simulink model "hexGroundContact"  (R2024a)
settings: configuration reference "standardSILConfiguraitonParams" (kept outside this file)
libraries: matrix_library x3, simulink x1
settings Model: Creator=jerem  LastModifiedBy=jerem
settings ConfigSetRef: SourceName=standardSILConfiguraitonParams  SourceLocation=Base Workspace

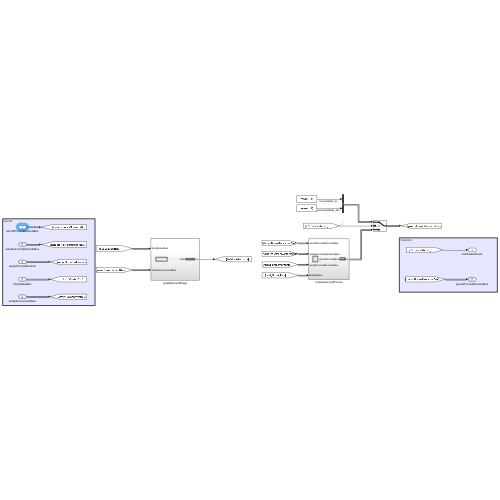
[thumbnail: Simulink's stored preview of the top-level diagram]
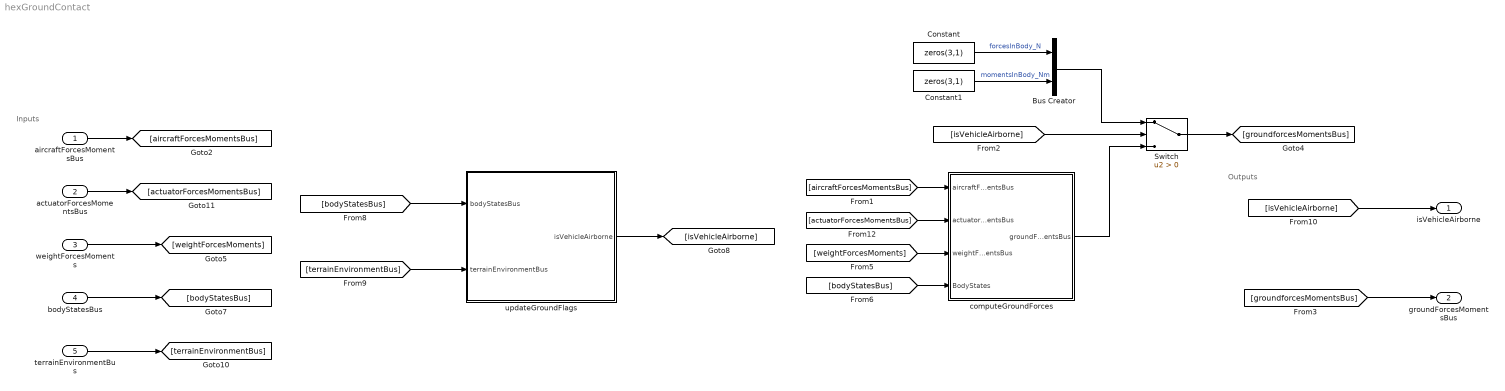
== system hexGroundContact ==
  note: Inputs
  note: Outputs
  aircraftForcesMomentsBus : Inport  OutDataTypeStr=Bus: AircraftForcesMomentsBus
  actuatorForcesMomentsBus : Inport  Port=2  OutDataTypeStr=Bus: ComponentForcesMomentsBus
  weightForcesMoments : Inport  Port=3  OutDataTypeStr=Bus: ComponentForcesMomentsBus
  bodyStatesBus : Inport  Port=4  OutDataTypeStr=Bus: BodyStateBus
  terrainEnvironmentBus : Inport  Port=5  OutDataTypeStr=Bus: TerrainEnvironmentBus
  Bus Creator : BusCreator  Inputs=2  OutDataTypeStr=Bus: ComponentForcesMomentsBus
  Constant : Constant  Value=zeros(3,1)
  Constant1 : Constant  Value=zeros(3,1)
  Switch : Switch  Criteria=u2 > Threshold  SaturateOnIntegerOverflow=off  InputSameDT=off
  computeGroundForces : Subsystem
  updateGroundFlags : Subsystem
  isVehicleAirborne : Outport  OutDataTypeStr=boolean
  groundForcesMomentsBus : Outport  Port=2  OutDataTypeStr=Bus: ComponentForcesMomentsBus
  wires:
  bodyStatesBus/1 -> [bodyStatesBus]
  terrainEnvironmentBus/1 -> [terrainEnvironmentBus]
  weightForcesMoments/1 -> [weightForcesMoments]
  aircraftForcesMomentsBus/1 -> [aircraftForcesMomentsBus]
  actuatorForcesMomentsBus/1 -> [actuatorForcesMomentsBus]
  [groundforcesMomentsBus] -> groundForcesMomentsBus/1
  [isVehicleAirborne] -> isVehicleAirborne/1
  Switch/1 -> [groundforcesMomentsBus]
  Bus Creator/1 -> Switch/1
  Constant/1 -> Bus Creator/1  "forcesInBody_N"
  updateGroundFlags/1(isVehicleAirborne) -> [isVehicleAirborne]
  [aircraftForcesMomentsBus] -> computeGroundForces/1(aircraftForcesMomentsBus)
  [bodyStatesBus] -> computeGroundForces/4(BodyStates)
  [terrainEnvironmentBus] -> updateGroundFlags/2(terrainEnvironmentBus)
  Constant1/1 -> Bus Creator/2  "momentsInBody_Nm"
  [weightForcesMoments] -> computeGroundForces/3(weightForcesMomentsBus)
  [actuatorForcesMomentsBus] -> computeGroundForces/2(actuatorForcesMomentsBus)
  computeGroundForces/1(groundForcesMomentsBus) -> Switch/3
  [bodyStatesBus] -> updateGroundFlags/1(bodyStatesBus)
  [isVehicleAirborne] -> Switch/2

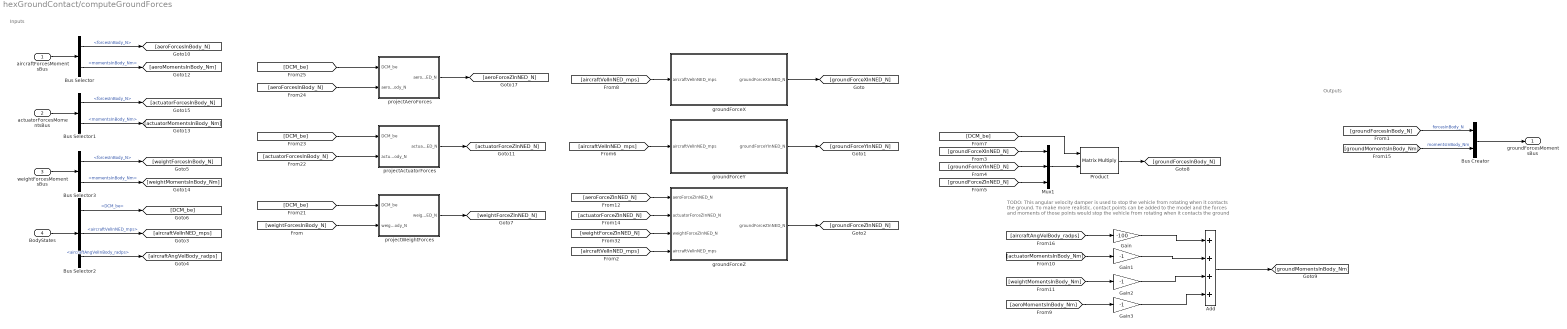
== system hexGroundContact/computeGroundForces ==
  note: Inputs
  note: Outputs
  note: TODO: This angular velocity damper is used to stop the vehicle from rotating when it contacts the ground. To make more realistic, contact points can be added to the model and the forces and moments of those points would stop the vehicle from rotating when it contacts the ground
  aircraftForcesMomentsBus : Inport  OutDataTypeStr=Bus: AircraftForcesMomentsBus
  actuatorForcesMomentsBus : Inport  Port=2  OutDataTypeStr=Bus: ComponentForcesMomentsBus
  weightForcesMomentsBus : Inport  Port=3  OutDataTypeStr=Bus: ComponentForcesMomentsBus
  BodyStates : Inport  Port=4  OutDataTypeStr=Bus: BodyStateBus
  Add : Sum  Inputs=++++
  Bus Creator : BusCreator  Inputs=2  OutDataTypeStr=Bus: ComponentForcesMomentsBus
  Bus Selector : BusSelector  OutputSignals=forcesInBody_N,momentsInBody_Nm
  Bus Selector1 : BusSelector  OutputSignals=forcesInBody_N,momentsInBody_Nm
  Bus Selector2 : BusSelector  OutputSignals=DCM_be,aircraftVelInNED_mps,aircraftAngVelInBody_radps
  Bus Selector3 : BusSelector  OutputSignals=forcesInBody_N,momentsInBody_Nm
  Gain : Gain  Gain=-100
  Gain1 : Gain  Gain=-1
  Gain2 : Gain  Gain=-1
  Gain3 : Gain  Gain=-1
  Mux1 : Mux  Inputs=3
  Product : Product  Multiplication=Matrix(*)
  groundForceX : Subsystem
  groundForceY : Subsystem
  groundForceZ : Subsystem
  projectActuatorForces : Subsystem
  projectAeroForces : Subsystem
  projectWeightForces : Subsystem
  groundForcesMomentsBus : Outport  OutDataTypeStr=Bus: ComponentForcesMomentsBus
  wires:
  aircraftForcesMomentsBus/1 -> Bus Selector/1
  groundForceX/1(groundForceXInNED_N) -> [groundForceXInNED_N]
  groundForceY/1(groundForceYInNED_N) -> [groundForceYInNED_N]
  groundForceZ/1(groundForceZInNED_N) -> [groundForceZInNED_N]
  [aeroForceZInNED_N] -> groundForceZ/1(aeroForceZInNED_N)
  [actuatorForceZInNED_N] -> groundForceZ/2(actuatorForceZInNED_N)
  [groundForceXInNED_N] -> Mux1/1
  [groundForceYInNED_N] -> Mux1/2
  [groundForceZInNED_N] -> Mux1/3
  Mux1/1 -> Product/2
  [DCM_be] -> Product/1
  actuatorForcesMomentsBus/1 -> Bus Selector1/1
  Bus Selector/1 -> [aeroForcesInBody_N]  "<forcesInBody_N>"
  BodyStates/1 -> Bus Selector2/1
  Bus Selector2/1 -> [DCM_be]  "<DCM_be>"
  [groundForcesInBody_N] -> Bus Creator/1  "forcesInBody_N"
  Product/1 -> [groundForcesInBody_N]
  weightForcesMomentsBus/1 -> Bus Selector3/1
  Bus Selector3/1 -> [weightForcesInBody_N]  "<forcesInBody_N>"
  [DCM_be] -> projectWeightForces/1(DCM_be)
  [weightForcesInBody_N] -> projectWeightForces/2(weightForcesInBody_N)
  projectWeightForces/1(weightForceZInNED_N) -> [weightForceZInNED_N]
  projectActuatorForces/1(actuatorForceZInNED_N) -> [actuatorForceZInNED_N]
  [actuatorForcesInBody_N] -> projectActuatorForces/2(actuatorForcesInBody_N)
  [DCM_be] -> projectActuatorForces/1(DCM_be)
  [DCM_be] -> projectAeroForces/1(DCM_be)
  [aeroForcesInBody_N] -> projectAeroForces/2(aeroForcesInBody_N)
  projectAeroForces/1(aeroForceZInNED_N) -> [aeroForceZInNED_N]
  Bus Selector1/1 -> [actuatorForcesInBody_N]  "<forcesInBody_N>"
  [weightForceZInNED_N] -> groundForceZ/3(weightForceZInNED_N)
  Bus Creator/1 -> groundForcesMomentsBus/1
  [groundMomentsInBody_Nm] -> Bus Creator/2  "momentsInBody_Nm"
  [aircraftVelInNED_mps] -> groundForceZ/4(aircraftVelInNED_mps)
  [aircraftVelInNED_mps] -> groundForceY/1(aircraftVelInNED_mps)
  [aircraftVelInNED_mps] -> groundForceX/1(aircraftVelInNED_mps)
  [aircraftAngVelBody_radps] -> Gain/1
  Gain/1 -> Add/1
  Add/1 -> [groundMomentsInBody_Nm]
  [actuatorMomentsInBody_Nm] -> Gain1/1
  [weightMomentsInBody_Nm] -> Gain2/1
  [aeroMomentsInBody_Nm] -> Gain3/1
  Gain1/1 -> Add/2
  Gain2/1 -> Add/3
  Gain3/1 -> Add/4
  Bus Selector/2 -> [aeroMomentsInBody_Nm]  "<momentsInBody_Nm>"
  Bus Selector1/2 -> [actuatorMomentsInBody_Nm]  "<momentsInBody_Nm>"
  Bus Selector3/2 -> [weightMomentsInBody_Nm]  "<momentsInBody_Nm>"
  Bus Selector2/2 -> [aircraftVelInNED_mps]  "<aircraftVelInNED_mps>"
  Bus Selector2/3 -> [aircraftAngVelBody_radps]  "<aircraftAngVelInBody_radps>"

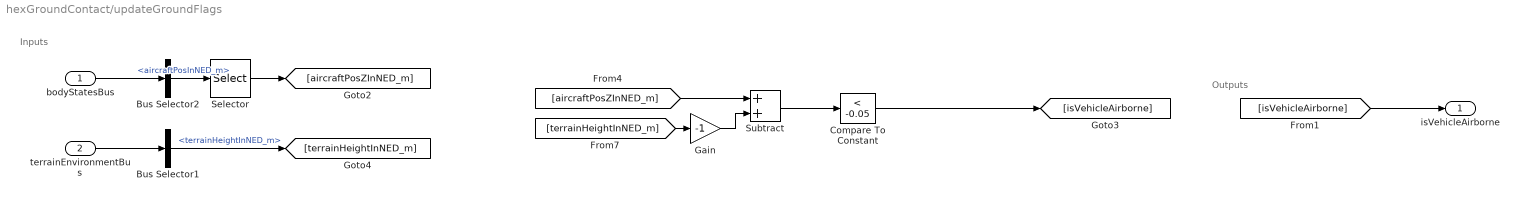
== system hexGroundContact/updateGroundFlags ==
  note: Outputs
  note: Inputs
  bodyStatesBus : Inport  OutDataTypeStr=Bus: BodyStateBus
  terrainEnvironmentBus : Inport  Port=2  OutDataTypeStr=Bus: TerrainEnvironmentBus
  Bus Selector1 : BusSelector  OutputSignals=terrainHeightInNED_m
  Bus Selector2 : BusSelector  OutputSignals=aircraftPosInNED_m
  Compare To Constant : simulink/Logic and Bit Operations/Compare To Constant  relop=<  const=-0.05  OutDataTypeStr=boolean
  Gain : Gain  Gain=-1
  Selector : Selector  InputPortWidth=3  IndexOptions=Index vector (dialog)  Indices=3  OutputSizes=1
  Subtract : Sum
  isVehicleAirborne : Outport  OutDataTypeStr=boolean
  wires:
  terrainEnvironmentBus/1 -> Bus Selector1/1
  bodyStatesBus/1 -> Bus Selector2/1
  Selector/1 -> [aircraftPosZInNED_m]
  [isVehicleAirborne] -> isVehicleAirborne/1
  Bus Selector1/1 -> [terrainHeightInNED_m]  "<terrainHeightInNED_m>"
  [aircraftPosZInNED_m] -> Subtract/1
  [terrainHeightInNED_m] -> Gain/1
  Subtract/1 -> Compare To Constant/1
  Gain/1 -> Subtract/2
  Bus Selector2/1 -> Selector/1  "<aircraftPosInNED_m>"
  Compare To Constant/1 -> [isVehicleAirborne]

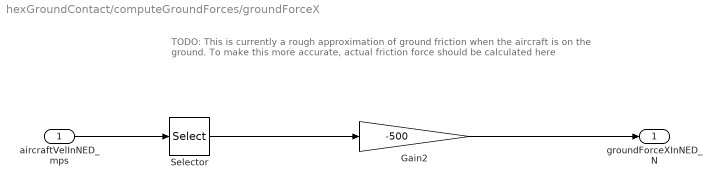
== system hexGroundContact/computeGroundForces/groundForceX ==
  note: TODO: This is currently a rough approximation of ground friction when the aircraft is on the ground. To make this more accurate, actual friction force should be calculated here
  aircraftVelInNED_mps : Inport
  Gain2 : Gain  Gain=-500
  Selector : Selector  InputPortWidth=3  IndexOptions=Index vector (dialog)  Indices=1  OutputSizes=1
  groundForceXInNED_N : Outport
  wires:
  aircraftVelInNED_mps/1 -> Selector/1
  Selector/1 -> Gain2/1
  Gain2/1 -> groundForceXInNED_N/1

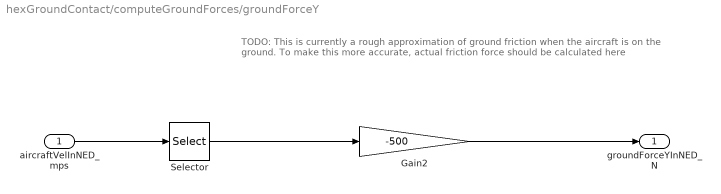
== system hexGroundContact/computeGroundForces/groundForceY ==
  note: TODO: This is currently a rough approximation of ground friction when the aircraft is on the ground. To make this more accurate, actual friction force should be calculated here
  aircraftVelInNED_mps : Inport
  Gain2 : Gain  Gain=-500
  Selector : Selector  InputPortWidth=3  IndexOptions=Index vector (dialog)  Indices=2  OutputSizes=1
  groundForceYInNED_N : Outport
  wires:
  Selector/1 -> Gain2/1
  aircraftVelInNED_mps/1 -> Selector/1
  Gain2/1 -> groundForceYInNED_N/1

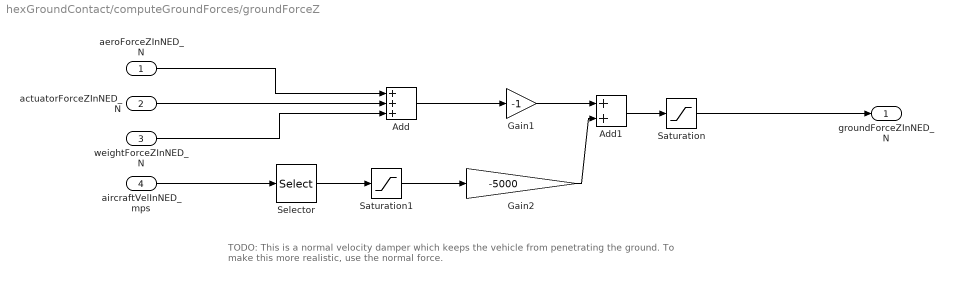
== system hexGroundContact/computeGroundForces/groundForceZ ==
  note: TODO: This is a normal velocity damper which keeps the vehicle from penetrating the ground. To make this more realistic, use the normal force.
  aeroForceZInNED_N : Inport
  actuatorForceZInNED_N : Inport  Port=2
  weightForceZInNED_N : Inport  Port=3
  aircraftVelInNED_mps : Inport  Port=4
  Add : Sum  Inputs=+++
  Add1 : Sum
  Gain1 : Gain  Gain=-1
  Gain2 : Gain  Gain=-5000
  Saturation : Saturate  UpperLimit=0  LowerLimit=-inf
  Saturation1 : Saturate  UpperLimit=inf  LowerLimit=0
  Selector : Selector  InputPortWidth=3  IndexOptions=Index vector (dialog)  Indices=3  OutputSizes=1
  groundForceZInNED_N : Outport
  wires:
  Add/1 -> Gain1/1
  aeroForceZInNED_N/1 -> Add/1
  actuatorForceZInNED_N/1 -> Add/2
  Gain1/1 -> Add1/1
  weightForceZInNED_N/1 -> Add/3
  Saturation/1 -> groundForceZInNED_N/1
  aircraftVelInNED_mps/1 -> Selector/1
  Selector/1 -> Saturation1/1
  Saturation1/1 -> Gain2/1
  Gain2/1 -> Add1/2
  Add1/1 -> Saturation/1

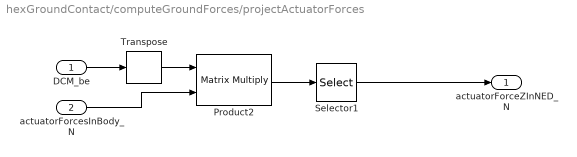
== system hexGroundContact/computeGroundForces/projectActuatorForces ==
  DCM_be : Inport
  actuatorForcesInBody_N : Inport  Port=2
  Product2 : Product  Multiplication=Matrix(*)
  Selector1 : Selector  InputPortWidth=3  IndexOptions=Index vector (dialog)  Indices=[3]  OutputSizes=1
  Transpose : matrix_library/Transpose
  actuatorForceZInNED_N : Outport
  wires:
  actuatorForcesInBody_N/1 -> Product2/2
  Product2/1 -> Selector1/1
  Selector1/1 -> actuatorForceZInNED_N/1
  DCM_be/1 -> Transpose/1
  Transpose/1 -> Product2/1

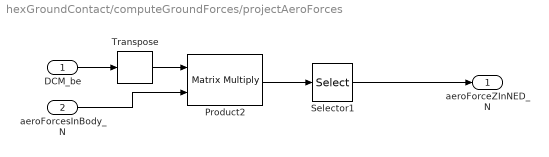
== system hexGroundContact/computeGroundForces/projectAeroForces ==
  DCM_be : Inport
  aeroForcesInBody_N : Inport  Port=2
  Product2 : Product  Multiplication=Matrix(*)
  Selector1 : Selector  InputPortWidth=3  IndexOptions=Index vector (dialog)  Indices=[3]  OutputSizes=1
  Transpose : matrix_library/Transpose
  aeroForceZInNED_N : Outport
  wires:
  Transpose/1 -> Product2/1
  DCM_be/1 -> Transpose/1
  Selector1/1 -> aeroForceZInNED_N/1
  Product2/1 -> Selector1/1
  aeroForcesInBody_N/1 -> Product2/2

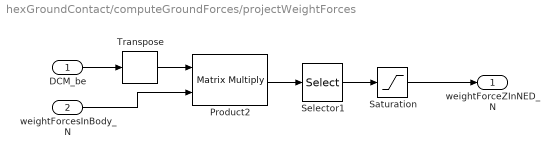
== system hexGroundContact/computeGroundForces/projectWeightForces ==
  DCM_be : Inport
  weightForcesInBody_N : Inport  Port=2
  Product2 : Product  Multiplication=Matrix(*)
  Saturation : Saturate  UpperLimit=Inf  LowerLimit=0
  Selector1 : Selector  InputPortWidth=3  IndexOptions=Index vector (dialog)  Indices=[3]  OutputSizes=1
  Transpose : matrix_library/Transpose
  weightForceZInNED_N : Outport
  wires:
  Transpose/1 -> Product2/1
  DCM_be/1 -> Transpose/1
  Saturation/1 -> weightForceZInNED_N/1
  Product2/1 -> Selector1/1
  Selector1/1 -> Saturation/1
  weightForcesInBody_N/1 -> Product2/2
